simulink model "Extended_Model_1_1"  (R2024a)
settings: Solver=ode15s  StartTime=0.0  StopTime=100  FixedStep=0.0001  MaxStep=0.01  RelTol=1e-3  AbsTol=1e-3  EnableMultiTasking=on
model workspace (MATLAB code in the model file):
  | F_load_x= 2e3; %[N]
  | F_load_y= 1e4; %[N]
  | 
  | d=0.01;   %[m]
  | l=1;      %[m]
  | L=l;      %[m] Node distance
  | H=L*cos(pi/6); %[m] Node distance
  | 
  | Density=7800; %[kg/m^3]
  | E=210;   %[GPa]
  | G=79;    %[GPa]
  | bm=0.01; %[1/s]  Default
  | bk=0.01; %[s] Default
  | 
  | b_rj=1; %[N*m*s/rad] Damp.Coef.Revolut joints
  | 
  | Size_frame=30; %[pixel]
undefined symbols (not defined in the file): F_x, F_y, X, Y, Z
libraries: sm_lib x317, nesl_utility x64, fl_lib x6, simulink x1
(part 1 of 9)
settings Model: NumberOfSteps=100000  Creator=Ing. Štefan Ondočko  LastModifiedBy=Ing. Štefan Ondočko
settings SolverCC: AutoScaleAbsTol=off  MaxZcPerStep=1
settings DataIOCC: LimitDataPoints=on  MaxDataPoints=10000  ReturnWorkspaceOutputs=off
settings OptimizationCC: ReuseModelBlockBuffer=off  LifeSpan=inf
settings DebuggingCC: UnconnectedInputMsg=warning  UnconnectedOutputMsg=warning  UnconnectedLineMsg=warning  AllowSymbolicDim=off  SubsystemReferenceDiagnosticForUnitTest=warning  SFUnexpectedBacktrackingDiag=warning  SFNoUnconditionalDefaultTransitionDiag=warning  SFExecutionAtInitializationDiag=none  ArithmeticOperatorsInVariantConditions=warning
settings ModelReferenceCC: EnableRefExpFcnMdlSchedulingChecks=on
settings SFSimCC: SimUseLocalCustomCode=off  CustomCodeUndefinedFunction=UseInterfaceOnly
settings RTWCC: RTWUseLocalCustomCode=off  GPUComputeCapability=3.5  DLArmComputeVersion=19.05
settings CodeAppCC: StateflowObjectComments=on
settings GRTTargetCC: TargetLangStandard=C89/C90 (ANSI)
settings ConfigComp: CovMetricSettings=dw  CovSaveCumulativeToWorkspaceVar=on  CovSaveSingleToWorkspaceVar=on  CovExternalEMLEnable=off  CovSFcnEnable=off
settings SimscapeCC: SimscapeLogType=all  SimscapeLogSimulationStatistics=on  SimscapeLogDataHistory=10000
settings ExplorerConfigSet: InternalSimMechanicsExplorerSettings="<ExplorerConfiguration><canonicalview>default</canonicalview><AnimationSetting><BasePlaybackSpeed>1.0</BasePlaybackSpeed><PlaybackSpeedFactor>2.0</PlaybackSpeedFactor></AnimationSetting><TilePanel><TileInfo><Tiles Columns=\"1\" Count=\"1\" Rows=\"1\"><Column Weight=\"1\"/><Row Weight=\"1\"/><Tile Height=\"1\" Width=\"1\" X=\"0\" Y=\"0\"/></Tiles></TileInfo><SceneInfo><SceneViewer><BGColor><R>1</R><G>1</G><B>1</B></BGColor><Camera><DoPerspective>off</DoPerspective><Position><X>1.34160017439744395</X><Y>2.43472426416735921</Y><Z>3.19868175252832421</Z></Position><Center><X>1.34160017439744395</X><Y>2.43472426416735921</Y><Z>1.1802899990698279e-08</Z></Center><Up><X>0</X><Y>1</Y><Z>-0</Z></Up><ViewLimDist>1</ViewLimDist><YLim>3.18022072065698147</YLim><XLim>1.97030216076793452</XLim></Camera></SceneViewer></SceneInfo></TilePanel><MechEditorPanel><Cameras/><GfxPanelCameraMap/><VideoCreator><PlaybackSpeedRatio>1.0</PlaybackSpeedRatio><FrameRate>30</FrameRate><VideoFormat>Motion JPEG AVI</VideoFormat><FrameSize>auto</FrameSize></VideoCreator></MechEditorPanel></ExplorerConfiguration>"

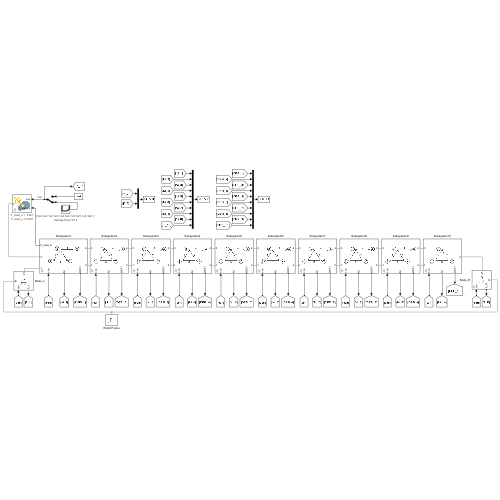
[thumbnail: Simulink's stored preview of the top-level diagram]
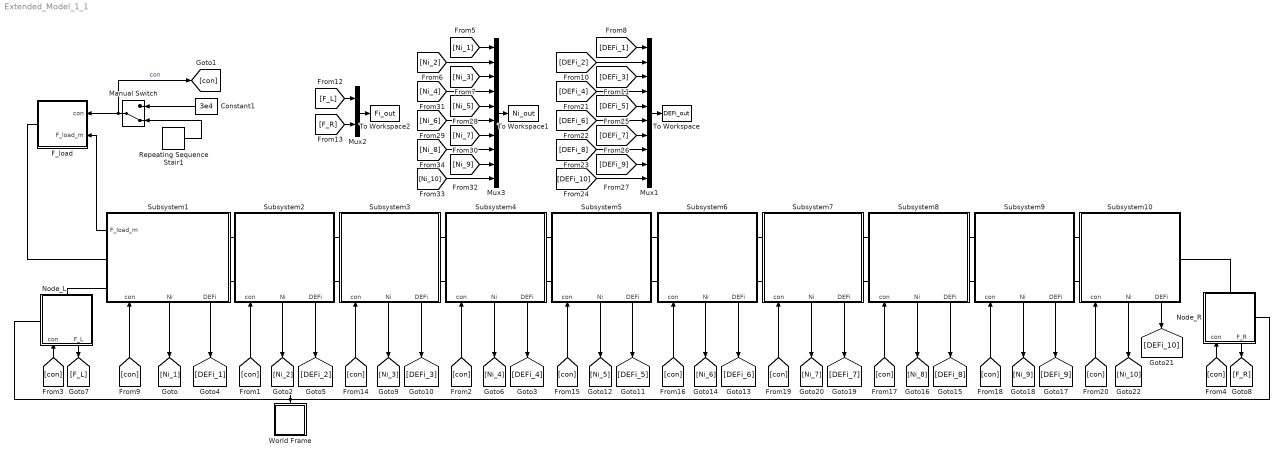
== system Extended_Model_1_1 ==
  Constant1 : Constant  Value=3e4
  F_load : Subsystem  mask{Fx=F_load_x, Fy=F_load_y, F=norm([F_x F_y])}
      mask prompts: Fx "Load Fx (N)"; Fy "Load Fy (N)"; F "Load F (N)"
      settings: AttributesFormatString=|
      | %<Fx> =  2 kN
      | %<Fy> =10 kN
      mask Display: image('D:sila_F.png');
  Manual Switch : ManualSwitch  CurrentSetting=0
  Mux1 : Mux  Inputs=10
  Mux2 : Mux  Inputs=2
  Mux3 : Mux  Inputs=10
  Node_L : Subsystem
      settings: PortSchema="{\"entries\":[{\"content\":{\"sides\":[{\"content\":{\"connectorIds\":[\"LConn1\"]},\"type\":\"ConnectorPlacement.EquallySpacedRectSide\",\"uuid\":\"d437545a-b6cd-405c-92f5-dfd428dd316c\"},{\"content\":{\"side\":\"RIGHT\"},\"type\":\"ConnectorPlacement.EquallySpacedRectSide\",\"uuid\":\"a6c866cb-015a-4ba6-a725-1ad5f0a48a96\"},{\"content\":{\"connectorIds\":[\"In1\",\"Out1\"],\"side\":\"TOP\"},\"type\":\"ConnectorPlacement.EquallySpacedRectSide\",\"uuid\":\"8c34f49c-4b46-4dd5-857b-cc1f00e0721b\"},{\"content\":{\"connectorIds\":[\"RConn1\"],\"side\":\"BOTTOM\"},\"type\":\"ConnectorPlacement.EquallySpacedRectSide\",\"uuid\":\"e1836308-c472-4635-822e-d84e1319bcc1\"}]},\"type\":\"ConnectorPlacement.EquallySpacedConnector\",\"uuid\":\"28d0e514-5749-47ac-8c9d-469c58f8fea4\"}],\"packageUris\":[\"http://schema.mathworks.com/mf0/Connector/R2020b\"],\"version\":\"1.0\"}"
  Node_R : Subsystem  mask{Nod2x=10*L}
      mask prompts: Nod2x "Nod2_offset_x"
      settings: PortSchema="{\"entries\":[{\"content\":{\"sides\":[{\"content\":{},\"type\":\"ConnectorPlacement.EquallySpacedRectSide\",\"uuid\":\"c52cac6f-2005-4bfe-89ae-e2a0406bbacd\"},{\"content\":{\"connectorIds\":[\"RConn1\"],\"side\":\"RIGHT\"},\"type\":\"ConnectorPlacement.EquallySpacedRectSide\",\"uuid\":\"5ceadddb-1bc3-405b-9850-d33e8ff0b50d\"},{\"content\":{\"connectorIds\":[\"In1\",\"Out1\"],\"side\":\"TOP\"},\"type\":\"ConnectorPlacement.EquallySpacedRectSide\",\"uuid\":\"947f3bae-c8fa-4b23-8ea1-709fee7d1677\"},{\"content\":{\"connectorIds\":[\"RConn2\"],\"side\":\"BOTTOM\"},\"type\":\"ConnectorPlacement.EquallySpacedRectSide\",\"uuid\":\"f9cd605e-29e4-49b7-a86d-9958a73b4d00\"}]},\"type\":\"ConnectorPlacement.EquallySpacedConnector\",\"uuid\":\"8856fa92-01df-438d-a79d-88950b3b721b\"}],\"packageUris\":[\"http://schema.mathworks.com/mf0/Connector/R2020b\"],\"version\":\"1.0\"}"
  Repeating Sequence Stair1 : simulink/Sources/Repeating Sequence Stair  OutValues=[1e2 3e2 1e3 3e3 1e4 3e4 1e5 3e5 1e6 3e6 ].'  tsamp=10  OutMin=[]  OutMax=[]  OutDataTypeStr=double  OutputDataTypeScalingMode=double  OutDataType=fixdt(0,8)  ConRadixGroup=Best Precision: Vector-wise  OutScaling=2^-12
      settings: AttributesFormatString=|
      | %<OutValues>
      | SampleTime=%<tsamp> s
  Subsystem1 : Subsystem  mask{Nod2x=-L, Nod3x=-L/2}
      mask prompts: Nod2x "Nod2_offset_x"; Nod3x "Nod3_offset_x"
      settings: PortSchema="{\"entries\":[{\"content\":{\"sides\":[{\"content\":{\"connectorIds\":[\"Out3\",\"LConn1\",\"LConn2\"]},\"type\":\"ConnectorPlacement.EquallySpacedRectSide\",\"uuid\":\"5b691ec6-fd17-4a8f-b07c-565e148aea54\"},{\"content\":{\"connectorIds\":[\"RConn1\",\"RConn2\"],\"side\":\"RIGHT\"},\"type\":\"ConnectorPlacement.EquallySpacedRectSide\",\"uuid\":\"123b4379-6f63-4bac-8b3e-d1a87a3d78c4\"},{\"content\":{\"side\":\"TOP\"},\"type\":\"ConnectorPlacement.EquallySpacedRectSide\",\"uuid\":\"f23bc5ee-4338-4010-a2a0-3e317780f82e\"},{\"content\":{\"connectorIds\":[\"In1\",\"Out1\",\"Out2\"],\"side\":\"BOTTOM\"},\"type\":\"ConnectorPlacement.EquallySpacedRectSide\",\"uuid\":\"f7fe3d2e-1943-42ac-96b9-26c8fbdc1d79\"}]},\"type\":\"ConnectorPlacement.EquallySpacedConnector\",\"uuid\":\"ed714cf3-4128-4128-8bb8-fa1b28911bdc\"}],\"packageUris\":[\"http://schema.mathworks.com/mf0/Connector/R2020b\"],\"version\":\"1.0\"}"
  Subsystem10 : Subsystem  mask{Nod2x=-10*L, Nod3x=-19*L/2}
      mask prompts: Nod2x "Nod2_offset_x"; Nod3x "Nod3_offset_x"
      settings: PortSchema="{\"entries\":[{\"content\":{\"sides\":[{\"content\":{\"connectorIds\":[\"LConn1\",\"LConn2\"]},\"type\":\"ConnectorPlacement.EquallySpacedRectSide\",\"uuid\":\"5b691ec6-fd17-4a8f-b07c-565e148aea54\"},{\"content\":{\"connectorIds\":[\"RConn1\"],\"side\":\"RIGHT\"},\"type\":\"ConnectorPlacement.EquallySpacedRectSide\",\"uuid\":\"123b4379-6f63-4bac-8b3e-d1a87a3d78c4\"},{\"content\":{\"side\":\"TOP\"},\"type\":\"ConnectorPlacement.EquallySpacedRectSide\",\"uuid\":\"f23bc5ee-4338-4010-a2a0-3e317780f82e\"},{\"content\":{\"connectorIds\":[\"In1\",\"Out1\",\"Out2\"],\"side\":\"BOTTOM\"},\"type\":\"ConnectorPlacement.EquallySpacedRectSide\",\"uuid\":\"f7fe3d2e-1943-42ac-96b9-26c8fbdc1d79\"}]},\"type\":\"ConnectorPlacement.EquallySpacedConnector\",\"uuid\":\"ed714cf3-4128-4128-8bb8-fa1b28911bdc\"}],\"packageUris\":[\"http://schema.mathworks.com/mf0/Connector/R2020b\"],\"version\":\"1.0\"}"
  Subsystem2 : Subsystem  mask{Nod2x=-2*L, Nod3x=-3*L/2}
      mask prompts: Nod2x "Nod2_offset_x"; Nod3x "Nod3_offset_x"
      settings: PortSchema="{\"entries\":[{\"content\":{\"sides\":[{\"content\":{\"connectorIds\":[\"LConn1\",\"LConn2\"]},\"type\":\"ConnectorPlacement.EquallySpacedRectSide\",\"uuid\":\"5b691ec6-fd17-4a8f-b07c-565e148aea54\"},{\"content\":{\"connectorIds\":[\"RConn1\",\"RConn2\"],\"side\":\"RIGHT\"},\"type\":\"ConnectorPlacement.EquallySpacedRectSide\",\"uuid\":\"123b4379-6f63-4bac-8b3e-d1a87a3d78c4\"},{\"content\":{\"side\":\"TOP\"},\"type\":\"ConnectorPlacement.EquallySpacedRectSide\",\"uuid\":\"f23bc5ee-4338-4010-a2a0-3e317780f82e\"},{\"content\":{\"connectorIds\":[\"In1\",\"Out1\",\"Out2\"],\"side\":\"BOTTOM\"},\"type\":\"ConnectorPlacement.EquallySpacedRectSide\",\"uuid\":\"f7fe3d2e-1943-42ac-96b9-26c8fbdc1d79\"}]},\"type\":\"ConnectorPlacement.EquallySpacedConnector\",\"uuid\":\"ed714cf3-4128-4128-8bb8-fa1b28911bdc\"}],\"packageUris\":[\"http://schema.mathworks.com/mf0/Connector/R2020b\"],\"version\":\"1.0\"}"
  Subsystem3 : Subsystem  mask{Nod2x=-3*L, Nod3x=-5*L/2}
      mask prompts: Nod2x "Nod2_offset_x"; Nod3x "Nod3_offset_x"
      settings: PortSchema="{\"entries\":[{\"content\":{\"sides\":[{\"content\":{\"connectorIds\":[\"LConn1\",\"LConn2\"]},\"type\":\"ConnectorPlacement.EquallySpacedRectSide\",\"uuid\":\"5b691ec6-fd17-4a8f-b07c-565e148aea54\"},{\"content\":{\"connectorIds\":[\"RConn1\",\"RConn2\"],\"side\":\"RIGHT\"},\"type\":\"ConnectorPlacement.EquallySpacedRectSide\",\"uuid\":\"123b4379-6f63-4bac-8b3e-d1a87a3d78c4\"},{\"content\":{\"side\":\"TOP\"},\"type\":\"ConnectorPlacement.EquallySpacedRectSide\",\"uuid\":\"f23bc5ee-4338-4010-a2a0-3e317780f82e\"},{\"content\":{\"connectorIds\":[\"In1\",\"Out1\",\"Out2\"],\"side\":\"BOTTOM\"},\"type\":\"ConnectorPlacement.EquallySpacedRectSide\",\"uuid\":\"f7fe3d2e-1943-42ac-96b9-26c8fbdc1d79\"}]},\"type\":\"ConnectorPlacement.EquallySpacedConnector\",\"uuid\":\"ed714cf3-4128-4128-8bb8-fa1b28911bdc\"}],\"packageUris\":[\"http://schema.mathworks.com/mf0/Connector/R2020b\"],\"version\":\"1.0\"}"
  Subsystem4 : Subsystem  mask{Nod2x=-4*L, Nod3x=-7*L/2}
      mask prompts: Nod2x "Nod2_offset_x"; Nod3x "Nod3_offset_x"
      settings: PortSchema="{\"entries\":[{\"content\":{\"sides\":[{\"content\":{\"connectorIds\":[\"LConn1\",\"LConn2\"]},\"type\":\"ConnectorPlacement.EquallySpacedRectSide\",\"uuid\":\"5b691ec6-fd17-4a8f-b07c-565e148aea54\"},{\"content\":{\"connectorIds\":[\"RConn1\",\"RConn2\"],\"side\":\"RIGHT\"},\"type\":\"ConnectorPlacement.EquallySpacedRectSide\",\"uuid\":\"123b4379-6f63-4bac-8b3e-d1a87a3d78c4\"},{\"content\":{\"side\":\"TOP\"},\"type\":\"ConnectorPlacement.EquallySpacedRectSide\",\"uuid\":\"f23bc5ee-4338-4010-a2a0-3e317780f82e\"},{\"content\":{\"connectorIds\":[\"In1\",\"Out1\",\"Out2\"],\"side\":\"BOTTOM\"},\"type\":\"ConnectorPlacement.EquallySpacedRectSide\",\"uuid\":\"f7fe3d2e-1943-42ac-96b9-26c8fbdc1d79\"}]},\"type\":\"ConnectorPlacement.EquallySpacedConnector\",\"uuid\":\"ed714cf3-4128-4128-8bb8-fa1b28911bdc\"}],\"packageUris\":[\"http://schema.mathworks.com/mf0/Connector/R2020b\"],\"version\":\"1.0\"}"
  Subsystem5 : Subsystem  mask{Nod2x=-5*L, Nod3x=-9*L/2}
      mask prompts: Nod2x "Nod2_offset_x"; Nod3x "Nod3_offset_x"
      settings: PortSchema="{\"entries\":[{\"content\":{\"sides\":[{\"content\":{\"connectorIds\":[\"LConn1\",\"LConn2\"]},\"type\":\"ConnectorPlacement.EquallySpacedRectSide\",\"uuid\":\"5b691ec6-fd17-4a8f-b07c-565e148aea54\"},{\"content\":{\"connectorIds\":[\"RConn1\",\"RConn2\"],\"side\":\"RIGHT\"},\"type\":\"ConnectorPlacement.EquallySpacedRectSide\",\"uuid\":\"123b4379-6f63-4bac-8b3e-d1a87a3d78c4\"},{\"content\":{\"side\":\"TOP\"},\"type\":\"ConnectorPlacement.EquallySpacedRectSide\",\"uuid\":\"f23bc5ee-4338-4010-a2a0-3e317780f82e\"},{\"content\":{\"connectorIds\":[\"In1\",\"Out1\",\"Out2\"],\"side\":\"BOTTOM\"},\"type\":\"ConnectorPlacement.EquallySpacedRectSide\",\"uuid\":\"f7fe3d2e-1943-42ac-96b9-26c8fbdc1d79\"}]},\"type\":\"ConnectorPlacement.EquallySpacedConnector\",\"uuid\":\"ed714cf3-4128-4128-8bb8-fa1b28911bdc\"}],\"packageUris\":[\"http://schema.mathworks.com/mf0/Connector/R2020b\"],\"version\":\"1.0\"}"
  Subsystem6 : Subsystem  mask{Nod2x=-6*L, Nod3x=-11*L/2}
      mask prompts: Nod2x "Nod2_offset_x"; Nod3x "Nod3_offset_x"
      settings: PortSchema="{\"entries\":[{\"content\":{\"sides\":[{\"content\":{\"connectorIds\":[\"LConn1\",\"LConn2\"]},\"type\":\"ConnectorPlacement.EquallySpacedRectSide\",\"uuid\":\"5b691ec6-fd17-4a8f-b07c-565e148aea54\"},{\"content\":{\"connectorIds\":[\"RConn1\",\"RConn2\"],\"side\":\"RIGHT\"},\"type\":\"ConnectorPlacement.EquallySpacedRectSide\",\"uuid\":\"123b4379-6f63-4bac-8b3e-d1a87a3d78c4\"},{\"content\":{\"side\":\"TOP\"},\"type\":\"ConnectorPlacement.EquallySpacedRectSide\",\"uuid\":\"f23bc5ee-4338-4010-a2a0-3e317780f82e\"},{\"content\":{\"connectorIds\":[\"In1\",\"Out1\",\"Out2\"],\"side\":\"BOTTOM\"},\"type\":\"ConnectorPlacement.EquallySpacedRectSide\",\"uuid\":\"f7fe3d2e-1943-42ac-96b9-26c8fbdc1d79\"}]},\"type\":\"ConnectorPlacement.EquallySpacedConnector\",\"uuid\":\"ed714cf3-4128-4128-8bb8-fa1b28911bdc\"}],\"packageUris\":[\"http://schema.mathworks.com/mf0/Connector/R2020b\"],\"version\":\"1.0\"}"
  Subsystem7 : Subsystem  mask{Nod2x=-7*L, Nod3x=-13*L/2}
      mask prompts: Nod2x "Nod2_offset_x"; Nod3x "Nod3_offset_x"
      settings: PortSchema="{\"entries\":[{\"content\":{\"sides\":[{\"content\":{\"connectorIds\":[\"LConn1\",\"LConn2\"]},\"type\":\"ConnectorPlacement.EquallySpacedRectSide\",\"uuid\":\"5b691ec6-fd17-4a8f-b07c-565e148aea54\"},{\"content\":{\"connectorIds\":[\"RConn1\",\"RConn2\"],\"side\":\"RIGHT\"},\"type\":\"ConnectorPlacement.EquallySpacedRectSide\",\"uuid\":\"123b4379-6f63-4bac-8b3e-d1a87a3d78c4\"},{\"content\":{\"side\":\"TOP\"},\"type\":\"ConnectorPlacement.EquallySpacedRectSide\",\"uuid\":\"f23bc5ee-4338-4010-a2a0-3e317780f82e\"},{\"content\":{\"connectorIds\":[\"In1\",\"Out1\",\"Out2\"],\"side\":\"BOTTOM\"},\"type\":\"ConnectorPlacement.EquallySpacedRectSide\",\"uuid\":\"f7fe3d2e-1943-42ac-96b9-26c8fbdc1d79\"}]},\"type\":\"ConnectorPlacement.EquallySpacedConnector\",\"uuid\":\"ed714cf3-4128-4128-8bb8-fa1b28911bdc\"}],\"packageUris\":[\"http://schema.mathworks.com/mf0/Connector/R2020b\"],\"version\":\"1.0\"}"
  Subsystem8 : Subsystem  mask{Nod2x=-8*L, Nod3x=-15*L/2}
      mask prompts: Nod2x "Nod2_offset_x"; Nod3x "Nod3_offset_x"
      settings: PortSchema="{\"entries\":[{\"content\":{\"sides\":[{\"content\":{\"connectorIds\":[\"LConn1\",\"LConn2\"]},\"type\":\"ConnectorPlacement.EquallySpacedRectSide\",\"uuid\":\"5b691ec6-fd17-4a8f-b07c-565e148aea54\"},{\"content\":{\"connectorIds\":[\"RConn1\",\"RConn2\"],\"side\":\"RIGHT\"},\"type\":\"ConnectorPlacement.EquallySpacedRectSide\",\"uuid\":\"123b4379-6f63-4bac-8b3e-d1a87a3d78c4\"},{\"content\":{\"side\":\"TOP\"},\"type\":\"ConnectorPlacement.EquallySpacedRectSide\",\"uuid\":\"f23bc5ee-4338-4010-a2a0-3e317780f82e\"},{\"content\":{\"connectorIds\":[\"In1\",\"Out1\",\"Out2\"],\"side\":\"BOTTOM\"},\"type\":\"ConnectorPlacement.EquallySpacedRectSide\",\"uuid\":\"f7fe3d2e-1943-42ac-96b9-26c8fbdc1d79\"}]},\"type\":\"ConnectorPlacement.EquallySpacedConnector\",\"uuid\":\"ed714cf3-4128-4128-8bb8-fa1b28911bdc\"}],\"packageUris\":[\"http://schema.mathworks.com/mf0/Connector/R2020b\"],\"version\":\"1.0\"}"
  Subsystem9 : Subsystem  mask{Nod2x=-9*L, Nod3x=-17*L/2}
      mask prompts: Nod2x "Nod2_offset_x"; Nod3x "Nod3_offset_x"
      settings: PortSchema="{\"entries\":[{\"content\":{\"sides\":[{\"content\":{\"connectorIds\":[\"LConn1\",\"LConn2\"]},\"type\":\"ConnectorPlacement.EquallySpacedRectSide\",\"uuid\":\"5b691ec6-fd17-4a8f-b07c-565e148aea54\"},{\"content\":{\"connectorIds\":[\"RConn1\",\"RConn2\"],\"side\":\"RIGHT\"},\"type\":\"ConnectorPlacement.EquallySpacedRectSide\",\"uuid\":\"123b4379-6f63-4bac-8b3e-d1a87a3d78c4\"},{\"content\":{\"side\":\"TOP\"},\"type\":\"ConnectorPlacement.EquallySpacedRectSide\",\"uuid\":\"f23bc5ee-4338-4010-a2a0-3e317780f82e\"},{\"content\":{\"connectorIds\":[\"In1\",\"Out1\",\"Out2\"],\"side\":\"BOTTOM\"},\"type\":\"ConnectorPlacement.EquallySpacedRectSide\",\"uuid\":\"f7fe3d2e-1943-42ac-96b9-26c8fbdc1d79\"}]},\"type\":\"ConnectorPlacement.EquallySpacedConnector\",\"uuid\":\"ed714cf3-4128-4128-8bb8-fa1b28911bdc\"}],\"packageUris\":[\"http://schema.mathworks.com/mf0/Connector/R2020b\"],\"version\":\"1.0\"}"
  To Workspace : ToWorkspace  VariableName=DEFi_out  SampleTime=-1
      settings: Decimation=3
  To Workspace1 : ToWorkspace  VariableName=Ni_out  SampleTime=-1
      settings: Decimation=3
  To Workspace2 : ToWorkspace  VariableName=Fi_out  SampleTime=-1
      settings: Decimation=3
  World Frame : Subsystem
      settings: PortSchema="{\"entries\":[{\"content\":{\"sides\":[{\"content\":{},\"type\":\"ConnectorPlacement.EquallySpacedRectSide\",\"uuid\":\"6a8e21d3-b0b2-4758-a6c8-a7be5ecb73b9\"},{\"content\":{\"side\":\"RIGHT\"},\"type\":\"ConnectorPlacement.EquallySpacedRectSide\",\"uuid\":\"42798d98-bef9-4838-9935-056c1ef1235d\"},{\"content\":{\"connectorIds\":[\"LConn1\"],\"side\":\"TOP\"},\"type\":\"ConnectorPlacement.EquallySpacedRectSide\",\"uuid\":\"7c8f84cf-9fc0-4b00-b00b-766e511bcfac\"}]},\"type\":\"ConnectorPlacement.EquallySpacedConnector\",\"uuid\":\"93a5f294-2ff9-4ffa-a830-6e6e0d522148\"}],\"packageUris\":[\"http://schema.mathworks.com/mf0/Connector/R2020b\"],\"version\":\"1.0\"}"
  wires:
  [con] -> Subsystem1/1(con)
  [con] -> Subsystem2/1(con)
  [con] -> Node_L/1(con)
  [con] -> Node_R/1(con)
  Repeating Sequence Stair1/1 -> Manual Switch/2
  Constant1/1 -> Manual Switch/1
  Manual Switch/1 -> F_load/1(con), [con]  "con"
  Subsystem1/3(F_load_m) -> F_load/2(F_load_m)
  Subsystem1/1(Ni) -> [Ni_1]
  Subsystem2/1(Ni) -> [Ni_2]
  [Ni_1] -> Mux3/1
  [Ni_2] -> Mux3/2
  [Ni_3] -> Mux3/3
  Subsystem1/2(DEFi) -> [DEFi_1]
  Subsystem2/2(DEFi) -> [DEFi_2]
  [DEFi_2] -> Mux1/2
  [DEFi_1] -> Mux1/1
  [DEFi_3] -> Mux1/3
  Node_L/1(F_L) -> [F_L]
  Node_R/1(F_R) -> [F_R]
  [F_R] -> Mux2/2
  [F_L] -> Mux2/1
  Mux2/1 -> To Workspace2/1
  Mux1/1 -> To Workspace/1
  Subsystem3/1(Ni) -> [Ni_3]
  Subsystem3/2(DEFi) -> [DEFi_3]
  [con] -> Subsystem3/1(con)
  Subsystem4/1(Ni) -> [Ni_4]
  [con] -> Subsystem4/1(con)
  Subsystem4/2(DEFi) -> [DEFi_4]
  Subsystem5/1(Ni) -> [Ni_5]
  [con] -> Subsystem5/1(con)
  Subsystem5/2(DEFi) -> [DEFi_5]
  Subsystem6/1(Ni) -> [Ni_6]
  [con] -> Subsystem6/1(con)
  Subsystem6/2(DEFi) -> [DEFi_6]
  [con] -> Subsystem7/1(con)
  Subsystem7/1(Ni) -> [Ni_7]
  Subsystem7/2(DEFi) -> [DEFi_7]
  [con] -> Subsystem8/1(con)
  Subsystem8/2(DEFi) -> [DEFi_8]
  Subsystem8/1(Ni) -> [Ni_8]
  [con] -> Subsystem9/1(con)
  Subsystem9/1(Ni) -> [Ni_9]
  Subsystem9/2(DEFi) -> [DEFi_9]
  [con] -> Subsystem10/1(con)
  Subsystem10/1(Ni) -> [Ni_10]
  Subsystem10/2(DEFi) -> [DEFi_10]
  [DEFi_5] -> Mux1/5
  [DEFi_4] -> Mux1/4
  [DEFi_6] -> Mux1/6
  [DEFi_8] -> Mux1/8
  [DEFi_10] -> Mux1/10
  [DEFi_7] -> Mux1/7
  [DEFi_9] -> Mux1/9
  Mux3/1 -> To Workspace1/1
  [Ni_6] -> Mux3/6
  [Ni_4] -> Mux3/4
  [Ni_5] -> Mux3/5
  [Ni_7] -> Mux3/7
  [Ni_8] -> Mux3/8
  [Ni_10] -> Mux3/10
  [Ni_9] -> Mux3/9
  connections:
  Node_L/LConn1 -- World Frame/LConn1 -- Node_R/RConn1
  Subsystem1/LConn2 -- Node_L/RConn1
  Subsystem1/RConn1 -- Subsystem2/LConn1
  Subsystem1/RConn2 -- Subsystem2/LConn2
  Subsystem10/RConn1 -- Node_R/RConn2
  Subsystem1/LConn1 -- F_load/RConn1
  Subsystem3/LConn2 -- Subsystem2/RConn2
  Subsystem3/LConn1 -- Subsystem2/RConn1
  Subsystem4/LConn1 -- Subsystem3/RConn1
  Subsystem4/LConn2 -- Subsystem3/RConn2
  Subsystem5/LConn1 -- Subsystem4/RConn1
  Subsystem5/LConn2 -- Subsystem4/RConn2
  Subsystem6/LConn1 -- Subsystem5/RConn1
  Subsystem6/LConn2 -- Subsystem5/RConn2
  Subsystem8/LConn1 -- Subsystem7/RConn1
  Subsystem9/LConn1 -- Subsystem8/RConn1
  Subsystem9/LConn2 -- Subsystem8/RConn2
  Subsystem8/LConn2 -- Subsystem7/RConn2
  Subsystem7/LConn1 -- Subsystem6/RConn1
  Subsystem7/LConn2 -- Subsystem6/RConn2
  Subsystem9/RConn1 -- Subsystem10/LConn1
  Subsystem9/RConn2 -- Subsystem10/LConn2

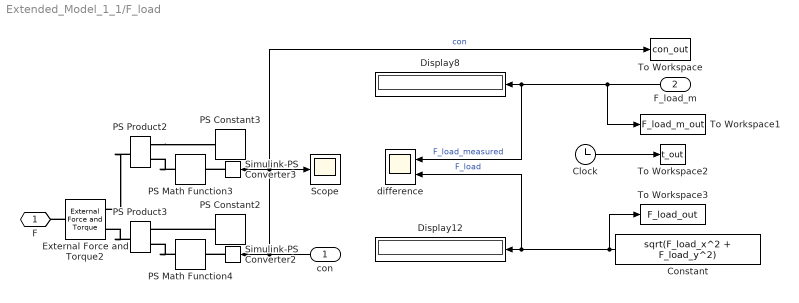
== system Extended_Model_1_1/F_load ==
  con : Inport
  F_load_m : Inport  Port=2
  Clock : Clock
  Constant : Constant  Value=sqrt(F_load_x^2 + F_load_y^2)
  Display12 : Display
      settings: Description=N  AttributesFormatString=%<Description>  Format=long_e
  Display8 : Display
      settings: Description=N  AttributesFormatString=%<Description>  Format=long_e
  External Force and Torque2 : sm_lib/Forces and Torques/External Force and Torque  EnableForceX=on  EnableForceY=on  EnableForceZ=off  EnableForce=off  ForceResolutionFrame=World  EnableTorqueX=off  EnableTorqueY=off  EnableTorqueZ=off  EnableTorque=off  TorqueResolutionFrame=AttachedFrame
  PS Constant2 : fl_lib/Physical Signals/Sources/PS Constant  constant=F_load_y
      settings: AttributesFormatString=%<constant>
  PS Constant3 : fl_lib/Physical Signals/Sources/PS Constant  constant=F_load_x
      settings: AttributesFormatString=%<constant>
  PS Math Function3 : fl_lib/Physical Signals/Functions/PS Math Function  fcn_choice=foundation.enum.math_function.reciprocal  v=1
  PS Math Function4 : fl_lib/Physical Signals/Functions/PS Math Function  fcn_choice=foundation.enum.math_function.reciprocal  v=1
  PS Product2 : fl_lib/Physical Signals/Functions/PS Product
  PS Product3 : fl_lib/Physical Signals/Functions/PS Product
  Scope : Scope
  Simulink-PS Converter2 : nesl_utility/Simulink-PS Converter  PhysicalDomain=network_engine_domain  SubClassName=ps_input  LeftPortType=input  RightPortType=output  PseudoPeriodic=off  Frequencies=[]  NoiseDistribution=none  NoiseParameters=[]  Unit=1  AffineConversion=off  FilteringAndDerivatives=provide  SimscapeFilterOrder=1  InputFilterTimeConstant=0.001  UdotUserProvided=0
  Simulink-PS Converter3 : nesl_utility/Simulink-PS Converter  PhysicalDomain=network_engine_domain  SubClassName=ps_input  LeftPortType=input  RightPortType=output  PseudoPeriodic=off  Frequencies=[]  NoiseDistribution=none  NoiseParameters=[]  Unit=1  AffineConversion=off  FilteringAndDerivatives=provide  SimscapeFilterOrder=1  InputFilterTimeConstant=0.001  UdotUserProvided=0
  To Workspace : ToWorkspace  VariableName=con_out  SampleTime=-1
  To Workspace1 : ToWorkspace  VariableName=F_load_m_out  SampleTime=-1
      settings: Decimation=3
  To Workspace2 : ToWorkspace  VariableName=t_out  SampleTime=-1
      settings: Decimation=3
  To Workspace3 : ToWorkspace  VariableName=F_load_out  SampleTime=-1
      settings: Decimation=3
  difference : Scope  NumInputPorts=2
  F : PMIOPort  Side=Right
  wires:
  F_load_m/1 -> To Workspace1/1, difference/1, Display8/1  "F_load_measured"
  Constant/1 -> To Workspace3/1, Display12/1, difference/2  "F_load"
  Clock/1 -> To Workspace2/1
  con/1 -> To Workspace/1, Scope/1, Simulink-PS Converter3/1, Simulink-PS Converter2/1  "con"
  connections:
  PS Math Function4/RConn1 -- PS Product3/LConn1
  Simulink-PS Converter2/RConn1 -- PS Math Function4/LConn1
  Simulink-PS Converter3/RConn1 -- PS Math Function3/LConn1
  PS Product2/LConn2 -- PS Constant3/RConn1
  PS Math Function3/RConn1 -- PS Product2/LConn1
  PS Constant2/RConn1 -- PS Product3/LConn2
  PS Product2/RConn1 -- External Force and Torque2/LConn1
  PS Product3/RConn1 -- External Force and Torque2/LConn2
  External Force and Torque2/RConn1 -- F/RConn1

== system Extended_Model_1_1/Node_L ==
  note: Node_L
  con : Inport
  Interpreted MATLAB Function : MATLABFcn  Description=u(1:2)  MATLABFcn=u(1:2)
      settings: AttributesFormatString=%<Description>
  PS-Simulink Converter1 : nesl_utility/PS-Simulink Converter  PhysicalDomain=network_engine_domain  SubClassName=ps_output  LeftPortType=input  RightPortType=output  PseudoPeriodic=off  Frequencies=[]  VectorFormat=inherit  Unit=1  AffineConversion=off
  Point : sm_lib/Curves and Surfaces/Point  Description=|  GraphicType=Marker  MarkerShape=Frame  MarkerSize=Size_frame  GraphicVisPropType=SimpleVisualProperties  GraphicDiffuseColor=[1 0 0]  GraphicOpacity=1.0  GraphicSpecularColor=[0.5 0.5 0.5 1.0]  GraphicAmbientColor=[0.15 0.15 0.15 1.0]  GraphicEmissiveColor=[0.0 0.0 0.0 1.0]  GraphicShininess=75
      | Frame
      | visualization
      settings: AttributesFormatString=%<Description>
  Point Cloud : sm_lib/Curves and Surfaces/Point Cloud  Description=|  CoordinatesMatrix=[0 0 0]  CoordinatesMatrixUnits=m  GraphicType=MarkerCloud  GraphicSphereRadius=d/2  GraphicSphereRadiusUnits=m  GraphicVisPropType=SimpleVisualProperties  GraphicDiffuseColor=[0.5 0.5 0.5]  GraphicOpacity=1  GraphicSpecularColor=[0.5 0.5 0.5 1.0]  GraphicAmbientColor=[0.15 0.15 0.15 1.0]  GraphicEmissiveColor=[0.0 0.0 0.0 1.0]  GraphicShininess=75
      | Graphic
      | sphere
      settings: AttributesFormatString=%<Description>
  Product : Product
  Revolute Joint1 : sm_lib/Joints/Revolute Joint  Description=|  JointMode=Normal  CompositeWrenchDir=FollowerOnBase  CompositeWrenchFrame=BaseFrame  SenseConstraintForce=off  SenseConstraintTorque=off  SenseTotalForce=on  SenseTotalTorque=off  PositionTargetSpecify=off  PositionTargetPriority=High  PositionTargetValue=10  PositionTargetValueUnits=deg  VelocityTargetSpecify=off  VelocityTargetPriority=High  VelocityTargetValue=0  VelocityTargetValueUnits=deg/s  EquilibriumPosition=0  EquilibriumPositionUnits=rad  SpringStiffness=0  SpringStiffnessUnits=N*m/rad  DampingCoefficient=b_rj  DampingCoefficientUnits=N*m*s/rad  LowerLimitSpecify=off  LowerLimitBound=-90  LowerLimitBoundUnits=deg  LowerLimitStiffness=1e4  LowerLimitStiffnessUnits=N*m/deg  LowerLimitDamping=10  LowerLimitDampingUnits=N*m/(deg/s)  LowerLimitTransitionRegionWidth=0.1  LowerLimitTransitionRegionWidthUnits=deg  UpperLimitSpecify=off  UpperLimitBound=90  UpperLimitBoundUnits=deg  UpperLimitStiffness=1e4  UpperLimitStiffnessUnits=N*m/deg  UpperLimitDamping=10  UpperLimitDampingUnits=N*m/(deg/s)  UpperLimitTransitionRegionWidth=0.1  UpperLimitTransitionRegionWidthUnits=deg  TorqueActuationMode=NoTorque  MotionActuationMode=ComputedMotion  SensePosition=off  SenseVelocity=off  SenseAcceleration=off  SenseTorqueForce=off  SenseLowerLimitTorqueForce=off  SenseUpperLimitTorqueForce=off
      | Total force
      | sensing
  B : PMIOPort  Side=Left
  F1 : PMIOPort  Port=2  Side=Right
  F_L : Outport
  wires:
  PS-Simulink Converter1/1 -> Interpreted MATLAB Function/1
  Interpreted MATLAB Function/1 -> Product/1
  Product/1 -> F_L/1
  con/1 -> Product/2
  connections:
  Point Cloud/LConn1 -- Revolute Joint1/RConn1 -- F1/RConn1
  PS-Simulink Converter1/LConn1 -- Revolute Joint1/RConn2
  Revolute Joint1/LConn1 -- Point/LConn1 -- B/RConn1

== system Extended_Model_1_1/Node_R ==
  note: Node_R
  con : Inport
  Interpreted MATLAB Function : MATLABFcn  Description=u(1:2)  MATLABFcn=u(1:2)
      settings: AttributesFormatString=%<Description>
  PS-Simulink Converter1 : nesl_utility/PS-Simulink Converter  PhysicalDomain=network_engine_domain  SubClassName=ps_output  LeftPortType=input  RightPortType=output  PseudoPeriodic=off  Frequencies=[]  VectorFormat=inherit  Unit=1  AffineConversion=off
  Point Cloud2 : sm_lib/Curves and Surfaces/Point Cloud  Description=|  CoordinatesMatrix=[0 0 0]  CoordinatesMatrixUnits=m  GraphicType=MarkerCloud  GraphicSphereRadius=d/2  GraphicSphereRadiusUnits=m  GraphicVisPropType=SimpleVisualProperties  GraphicDiffuseColor=[0.5 0.5 0.5]  GraphicOpacity=1  GraphicSpecularColor=[0.5 0.5 0.5 1.0]  GraphicAmbientColor=[0.15 0.15 0.15 1.0]  GraphicEmissiveColor=[0.0 0.0 0.0 1.0]  GraphicShininess=75
      | Graphic
      | sphere
      settings: AttributesFormatString=%<Description>
  Point1 : sm_lib/Curves and Surfaces/Point  Description=|  GraphicType=Marker  MarkerShape=Frame  MarkerSize=Size_frame  GraphicVisPropType=SimpleVisualProperties  GraphicDiffuseColor=[1 0 0]  GraphicOpacity=1.0  GraphicSpecularColor=[0.5 0.5 0.5 1.0]  GraphicAmbientColor=[0.15 0.15 0.15 1.0]  GraphicEmissiveColor=[0.0 0.0 0.0 1.0]  GraphicShininess=75
      | Frame
      | visualization
      settings: AttributesFormatString=%<Description>
  Product : Product
  Revolute Joint : sm_lib/Joints/Revolute Joint  JointMode=Normal  CompositeWrenchDir=FollowerOnBase  CompositeWrenchFrame=BaseFrame  SenseConstraintForce=off  SenseConstraintTorque=off  SenseTotalForce=on  SenseTotalTorque=off  PositionTargetSpecify=off  PositionTargetPriority=High  PositionTargetValue=0  PositionTargetValueUnits=deg  VelocityTargetSpecify=off  VelocityTargetPriority=High  VelocityTargetValue=0  VelocityTargetValueUnits=deg/s  EquilibriumPosition=0  EquilibriumPositionUnits=rad  SpringStiffness=0  SpringStiffnessUnits=N*m/rad  DampingCoefficient=b_rj  DampingCoefficientUnits=N*m*s/rad  LowerLimitSpecify=off  LowerLimitBound=-90  LowerLimitBoundUnits=deg  LowerLimitStiffness=1e4  LowerLimitStiffnessUnits=N*m/deg  LowerLimitDamping=10  LowerLimitDampingUnits=N*m/(deg/s)  LowerLimitTransitionRegionWidth=0.1  LowerLimitTransitionRegionWidthUnits=deg  UpperLimitSpecify=off  UpperLimitBound=90  UpperLimitBoundUnits=deg  UpperLimitStiffness=1e4  UpperLimitStiffnessUnits=N*m/deg  UpperLimitDamping=10  UpperLimitDampingUnits=N*m/(deg/s)  UpperLimitTransitionRegionWidth=0.1  UpperLimitTransitionRegionWidthUnits=deg  TorqueActuationMode=NoTorque  MotionActuationMode=ComputedMotion  SensePosition=off  SenseVelocity=off  SenseAcceleration=off  SenseTorqueForce=off  SenseLowerLimitTorqueForce=off  SenseUpperLimitTorqueForce=off
  Rigid Transform1 : sm_lib/Frames and Transforms/Rigid Transform  Description=Offset  RotationMethod=None  FollAlignAxisA=+X  BaseAlignAxisA=+Y  FollAlignAxisB=+Y  BaseAlignAxisB=+Z  RotationStandardAxis=+Z  RotationAngle=0.0  RotationAngleUnits=deg  RotationArbitraryAxis=[0 0 1]  RotationSequenceAxes=FollowerAxes  RotationSequence=XYX  RotationSequenceAngles=[0 0 0]  RotationSequenceAnglesUnits=deg  RotationMatrix=[1 0 0; 0 1 0; 0 0 1]  Quaternion=[1 0 0 0]  TranslationMethod=Cartesian  TranslationCartesianOffset=[Nod2x 0 0]  TranslationCartesianOffsetUnits=m  TranslationStandardAxis=+Z  TranslationStandardOffset=0  TranslationStandardOffsetUnits=m  TranslationROffset=0  TranslationROffsetUnits=m  TranslationThetaOffset=0  TranslationThetaOffsetUnits=deg  TranslationZOffset=0  TranslationZOffsetUnits=m
      settings: AttributesFormatString=|
      | %<Description>
      | %<TranslationCartesianOffset> %<TranslationCartesianOffsetUnits>
  B : PMIOPort  Side=Right
  F1 : PMIOPort  Port=2  Side=Right
  F_R : Outport
  wires:
  PS-Simulink Converter1/1 -> Interpreted MATLAB Function/1
  con/1 -> Product/2
  Product/1 -> F_R/1
  Interpreted MATLAB Function/1 -> Product/1
  connections:
  F1/RConn1 -- Point Cloud2/LConn1 -- Revolute Joint/RConn1
  Rigid Transform1/RConn1 -- Revolute Joint/LConn1 -- Point1/LConn1
  Revolute Joint/RConn2 -- PS-Simulink Converter1/LConn1
  Rigid Transform1/LConn1 -- B/RConn1

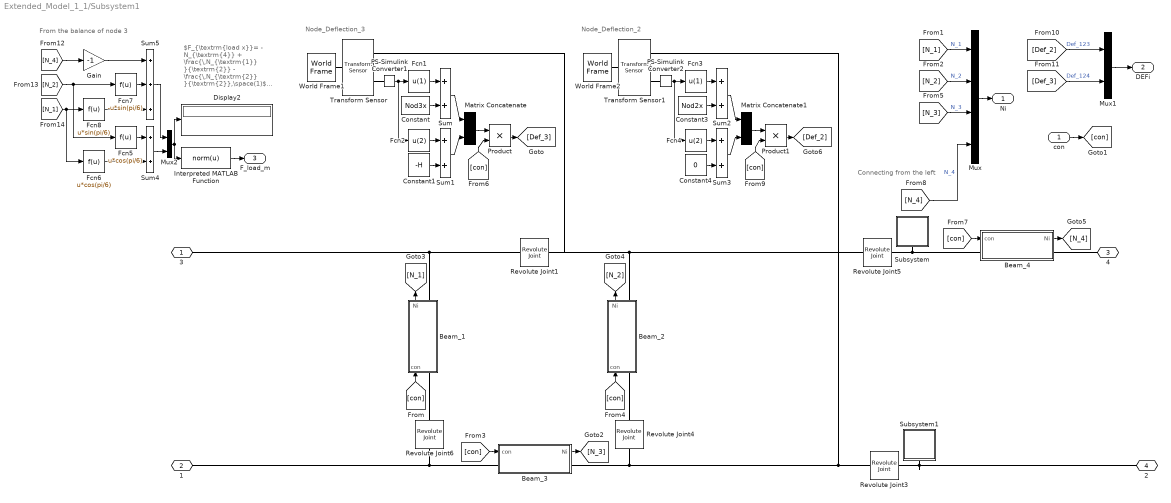
== system Extended_Model_1_1/Subsystem1 ==
  note: Connecting from the left
  note: Node_Deflection_3
  note: Node_Deflection_2
  note: $F_{\textrm{load x}}= - N_{\textrm{4}} + \frac{\,N_{\textrm{1}} }{\textrm{2}} - \frac{\,N_{\textrm{2}} }{\textrm{2}},\space(1)$
      | $F_{\textrm{load y}}=\frac{\sqrt{3}\,N_1 }{2} + \frac{\sqrt{3}\,N_2 }{2},\space(2)$
  note: From the balance of node 3
  con : Inport
  Beam_1 : Subsystem
  Beam_2 : Subsystem
  Beam_3 : Subsystem
  Beam_4 : Subsystem
  Constant : Constant  Value=Nod3x
  Constant1 : Constant  Value=-H
  Constant3 : Constant  Value=Nod2x
  Constant4 : Constant  Value=0
  Display2 : Display
      settings: Description=N  AttributesFormatString=%<Description>  Format=long_e
  Fcn1 : Fcn  Expr=u(1)
  Fcn2 : Fcn  Expr=u(2)
  Fcn3 : Fcn  Expr=u(1)
  Fcn4 : Fcn  Expr=u(2)
  Fcn5 : Fcn  Description=-u/sqrt(2)  Expr=u*cos(pi/6)
      settings: AttributesFormatString=%<Expr>
  Fcn6 : Fcn  Description=-u/sqrt(2)  Expr=u*cos(pi/6)
      settings: AttributesFormatString=%<Expr>
  Fcn7 : Fcn  Description=-u/sqrt(2)  Expr=-u*sin(pi/6)
      settings: AttributesFormatString=%<Expr>
  Fcn8 : Fcn  Description=-u/sqrt(2)  Expr=u*sin(pi/6)
      settings: AttributesFormatString=%<Expr>
  Gain : Gain  Gain=-1
  Interpreted MATLAB Function : MATLABFcn  Description=Norm  MATLABFcn=norm(u)
      settings: AttributesFormatString=%<Description>
  Matrix Concatenate : Concatenate  ConcatenateDimension=2
      settings: AttributesFormatString=%<Description>
  Matrix Concatenate1 : Concatenate  ConcatenateDimension=2
      settings: AttributesFormatString=%<Description>
  Mux : Mux
  Mux1 : Mux  Inputs=2
  Mux2 : Mux  Inputs=2
  PS-Simulink Converter1 : nesl_utility/PS-Simulink Converter  PhysicalDomain=network_engine_domain  SubClassName=ps_output  LeftPortType=input  RightPortType=output  PseudoPeriodic=off  Frequencies=[]  VectorFormat=inherit  Unit=1  AffineConversion=off
  PS-Simulink Converter2 : nesl_utility/PS-Simulink Converter  PhysicalDomain=network_engine_domain  SubClassName=ps_output  LeftPortType=input  RightPortType=output  PseudoPeriodic=off  Frequencies=[]  VectorFormat=inherit  Unit=1  AffineConversion=off
  Product : Product
  Product1 : Product
  Revolute Joint1 : sm_lib/Joints/Revolute Joint  JointMode=Normal  CompositeWrenchDir=FollowerOnBase  CompositeWrenchFrame=BaseFrame  SenseConstraintForce=off  SenseConstraintTorque=off  SenseTotalForce=off  SenseTotalTorque=off  PositionTargetSpecify=on  PositionTargetPriority=Low  PositionTargetValue=pi/3  PositionTargetValueUnits=rad  VelocityTargetSpecify=off  VelocityTargetPriority=High  VelocityTargetValue=0  VelocityTargetValueUnits=deg/s  EquilibriumPosition=0  EquilibriumPositionUnits=rad  SpringStiffness=0  SpringStiffnessUnits=N*m/rad  DampingCoefficient=b_rj  DampingCoefficientUnits=N*m*s/rad  LowerLimitSpecify=off  LowerLimitBound=-90  LowerLimitBoundUnits=deg  LowerLimitStiffness=1e4  LowerLimitStiffnessUnits=N*m/deg  LowerLimitDamping=10  LowerLimitDampingUnits=N*m/(deg/s)  LowerLimitTransitionRegionWidth=0.1  LowerLimitTransitionRegionWidthUnits=deg  UpperLimitSpecify=off  UpperLimitBound=90  UpperLimitBoundUnits=deg  UpperLimitStiffness=1e4  UpperLimitStiffnessUnits=N*m/deg  UpperLimitDamping=10  UpperLimitDampingUnits=N*m/(deg/s)  UpperLimitTransitionRegionWidth=0.1  UpperLimitTransitionRegionWidthUnits=deg  TorqueActuationMode=NoTorque  MotionActuationMode=ComputedMotion  SensePosition=off  SenseVelocity=off  SenseAcceleration=off  SenseTorqueForce=off  SenseLowerLimitTorqueForce=off  SenseUpperLimitTorqueForce=off
      settings: AttributesFormatString=%<PositionTargetValue>
  Revolute Joint3 : sm_lib/Joints/Revolute Joint  JointMode=Normal  CompositeWrenchDir=FollowerOnBase  CompositeWrenchFrame=BaseFrame  SenseConstraintForce=off  SenseConstraintTorque=off  SenseTotalForce=off  SenseTotalTorque=off  PositionTargetSpecify=on  PositionTargetPriority=Low  PositionTargetValue=0  PositionTargetValueUnits=rad  VelocityTargetSpecify=off  VelocityTargetPriority=High  VelocityTargetValue=0  VelocityTargetValueUnits=deg/s  EquilibriumPosition=0  EquilibriumPositionUnits=rad  SpringStiffness=0  SpringStiffnessUnits=N*m/rad  DampingCoefficient=b_rj  DampingCoefficientUnits=N*m*s/rad  LowerLimitSpecify=off  LowerLimitBound=-90  LowerLimitBoundUnits=deg  LowerLimitStiffness=1e4  LowerLimitStiffnessUnits=N*m/deg  LowerLimitDamping=10  LowerLimitDampingUnits=N*m/(deg/s)  LowerLimitTransitionRegionWidth=0.1  LowerLimitTransitionRegionWidthUnits=deg  UpperLimitSpecify=off  UpperLimitBound=90  UpperLimitBoundUnits=deg  UpperLimitStiffness=1e4  UpperLimitStiffnessUnits=N*m/deg  UpperLimitDamping=10  UpperLimitDampingUnits=N*m/(deg/s)  UpperLimitTransitionRegionWidth=0.1  UpperLimitTransitionRegionWidthUnits=deg  TorqueActuationMode=NoTorque  MotionActuationMode=ComputedMotion  SensePosition=off  SenseVelocity=off  SenseAcceleration=off  SenseTorqueForce=off  SenseLowerLimitTorqueForce=off  SenseUpperLimitTorqueForce=off
      settings: AttributesFormatString=%<PositionTargetValue>
  Revolute Joint4 : sm_lib/Joints/Revolute Joint  JointMode=Normal  CompositeWrenchDir=FollowerOnBase  CompositeWrenchFrame=BaseFrame  SenseConstraintForce=off  SenseConstraintTorque=off  SenseTotalForce=off  SenseTotalTorque=off  PositionTargetSpecify=off  PositionTargetPriority=High  PositionTargetValue=0  PositionTargetValueUnits=deg  VelocityTargetSpecify=off  VelocityTargetPriority=High  VelocityTargetValue=0  VelocityTargetValueUnits=deg/s  EquilibriumPosition=0  EquilibriumPositionUnits=rad  SpringStiffness=0  SpringStiffnessUnits=N*m/rad  DampingCoefficient=b_rj  DampingCoefficientUnits=N*m*s/rad  LowerLimitSpecify=off  LowerLimitBound=-90  LowerLimitBoundUnits=deg  LowerLimitStiffness=1e4  LowerLimitStiffnessUnits=N*m/deg  LowerLimitDamping=10  LowerLimitDampingUnits=N*m/(deg/s)  LowerLimitTransitionRegionWidth=0.1  LowerLimitTransitionRegionWidthUnits=deg  UpperLimitSpecify=off  UpperLimitBound=90  UpperLimitBoundUnits=deg  UpperLimitStiffness=1e4  UpperLimitStiffnessUnits=N*m/deg  UpperLimitDamping=10  UpperLimitDampingUnits=N*m/(deg/s)  UpperLimitTransitionRegionWidth=0.1  UpperLimitTransitionRegionWidthUnits=deg  TorqueActuationMode=NoTorque  MotionActuationMode=ComputedMotion  SensePosition=off  SenseVelocity=off  SenseAcceleration=off  SenseTorqueForce=off  SenseLowerLimitTorqueForce=off  SenseUpperLimitTorqueForce=off
  Revolute Joint5 : sm_lib/Joints/Revolute Joint  JointMode=Normal  CompositeWrenchDir=FollowerOnBase  CompositeWrenchFrame=BaseFrame  SenseConstraintForce=off  SenseConstraintTorque=off  SenseTotalForce=off  SenseTotalTorque=off  PositionTargetSpecify=on  PositionTargetPriority=Low  PositionTargetValue=-4*pi/6  PositionTargetValueUnits=rad  VelocityTargetSpecify=off  VelocityTargetPriority=High  VelocityTargetValue=0  VelocityTargetValueUnits=deg/s  EquilibriumPosition=0  EquilibriumPositionUnits=rad  SpringStiffness=0  SpringStiffnessUnits=N*m/rad  DampingCoefficient=b_rj  DampingCoefficientUnits=N*m*s/rad  LowerLimitSpecify=off  LowerLimitBound=-90  LowerLimitBoundUnits=deg  LowerLimitStiffness=1e4  LowerLimitStiffnessUnits=N*m/deg  LowerLimitDamping=10  LowerLimitDampingUnits=N*m/(deg/s)  LowerLimitTransitionRegionWidth=0.1  LowerLimitTransitionRegionWidthUnits=deg  UpperLimitSpecify=off  UpperLimitBound=90  UpperLimitBoundUnits=deg  UpperLimitStiffness=1e4  UpperLimitStiffnessUnits=N*m/deg  UpperLimitDamping=10  UpperLimitDampingUnits=N*m/(deg/s)  UpperLimitTransitionRegionWidth=0.1  UpperLimitTransitionRegionWidthUnits=deg  TorqueActuationMode=NoTorque  MotionActuationMode=ComputedMotion  SensePosition=off  SenseVelocity=off  SenseAcceleration=off  SenseTorqueForce=off  SenseLowerLimitTorqueForce=off  SenseUpperLimitTorqueForce=off
      settings: AttributesFormatString=%<PositionTargetValue>
  Revolute Joint6 : sm_lib/Joints/Revolute Joint  JointMode=Normal  CompositeWrenchDir=FollowerOnBase  CompositeWrenchFrame=BaseFrame  SenseConstraintForce=off  SenseConstraintTorque=off  SenseTotalForce=off  SenseTotalTorque=off  PositionTargetSpecify=on  PositionTargetPriority=Low  PositionTargetValue=pi/3  PositionTargetValueUnits=rad  VelocityTargetSpecify=off  VelocityTargetPriority=High  VelocityTargetValue=0  VelocityTargetValueUnits=deg/s  EquilibriumPosition=0  EquilibriumPositionUnits=rad  SpringStiffness=0  SpringStiffnessUnits=N*m/rad  DampingCoefficient=b_rj  DampingCoefficientUnits=N*m*s/rad  LowerLimitSpecify=off  LowerLimitBound=-90  LowerLimitBoundUnits=deg  LowerLimitStiffness=1e4  LowerLimitStiffnessUnits=N*m/deg  LowerLimitDamping=10  LowerLimitDampingUnits=N*m/(deg/s)  LowerLimitTransitionRegionWidth=0.1  LowerLimitTransitionRegionWidthUnits=deg  UpperLimitSpecify=off  UpperLimitBound=90  UpperLimitBoundUnits=deg  UpperLimitStiffness=1e4  UpperLimitStiffnessUnits=N*m/deg  UpperLimitDamping=10  UpperLimitDampingUnits=N*m/(deg/s)  UpperLimitTransitionRegionWidth=0.1  UpperLimitTransitionRegionWidthUnits=deg  TorqueActuationMode=NoTorque  MotionActuationMode=ComputedMotion  SensePosition=off  SenseVelocity=off  SenseAcceleration=off  SenseTorqueForce=off  SenseLowerLimitTorqueForce=off  SenseUpperLimitTorqueForce=off
      settings: AttributesFormatString=%<PositionTargetValue>
  Subsystem : Subsystem
  Subsystem1 : Subsystem
  Sum{,1..3} (4 alike) : Sum  Inputs=2
  Sum4 : Sum
  Sum5 : Sum  Inputs=3
  Transform Sensor : sm_lib/Frames and Transforms/Transform Sensor  Description=|  MeasurementFrame=World  RotationSequence=XYX  SenseAngle=off  SenseAxis=off  SenseQ=off  SenseR=off  SenseRotationSequence=off  SenseOmegaX=off  SenseOmegaY=off  SenseOmegaZ=off  SenseOmega=off  SenseQDot=off  SenseRDot=off  SenseRotationSequenceDot=off  SenseAlphaX=off  SenseAlphaY=off  SenseAlphaZ=off  SenseAlpha=off  SenseQDDot=off  SenseRDDot=off  SenseX=off  SenseY=off  SenseZ=off  SenseXYZ=on  SenseRad=off  SenseAzim=off  SenseDist=off  SenseInc=off  SenseXDot=off  SenseYDot=off  SenseZDot=off  SenseXYZDot=off  SenseRadDot=off  SenseAzimDot=off  SenseDistDot=off  SenseIncDot=off  SenseXDDot=off  SenseYDDot=off  SenseZDDot=off  SenseXYZDDot=off  SenseRadDDot=off  SenseAzimDDot=off  SenseDistDDot=off  SenseIncDDot=off
      | Translation
      | [x, y, z]
      settings: AttributesFormatString=%<Description>
  Transform Sensor1 : sm_lib/Frames and Transforms/Transform Sensor  Description=|  MeasurementFrame=World  RotationSequence=XYX  SenseAngle=off  SenseAxis=off  SenseQ=off  SenseR=off  SenseRotationSequence=off  SenseOmegaX=off  SenseOmegaY=off  SenseOmegaZ=off  SenseOmega=off  SenseQDot=off  SenseRDot=off  SenseRotationSequenceDot=off  SenseAlphaX=off  SenseAlphaY=off  SenseAlphaZ=off  SenseAlpha=off  SenseQDDot=off  SenseRDDot=off  SenseX=off  SenseY=off  SenseZ=off  SenseXYZ=on  SenseRad=off  SenseAzim=off  SenseDist=off  SenseInc=off  SenseXDot=off  SenseYDot=off  SenseZDot=off  SenseXYZDot=off  SenseRadDot=off  SenseAzimDot=off  SenseDistDot=off  SenseIncDot=off  SenseXDDot=off  SenseYDDot=off  SenseZDDot=off  SenseXYZDDot=off  SenseRadDDot=off  SenseAzimDDot=off  SenseDistDDot=off  SenseIncDDot=off
      | Translation
      | [x, y, z]
      settings: AttributesFormatString=%<Description>
  World Frame1 : sm_lib/Frames and Transforms/World Frame
  World Frame2 : sm_lib/Frames and Transforms/World Frame
  3 : PMIOPort  Side=Left
  1 : PMIOPort  Port=2  Side=Left
  4 : PMIOPort  Port=3  Side=Right
  2 : PMIOPort  Port=4  Side=Right
  Ni : Outport
  DEFi : Outport  Port=2
  F_load_m : Outport  Port=3
  wires:
  Sum2/1 -> Matrix Concatenate1/1
  Constant1/1 -> Sum1/2
  PS-Simulink Converter2/1 -> Fcn4/1, Fcn3/1
  Matrix Concatenate1/1 -> Product1/1
  [N_2] -> Mux/2  "N_2"
  Fcn1/1 -> Sum/1
  PS-Simulink Converter1/1 -> Fcn2/1, Fcn1/1
  [N_4] -> Mux/4  "N_4"
  Mux1/1 -> DEFi/1
  Beam_1/1(Ni) -> [N_1]
  [con] -> Beam_1/1(con)
  Beam_3/1(Ni) -> [N_3]
  [Def_2] -> Mux1/1  "Def_123"
  Constant/1 -> Sum/2
  [con] -> Product1/2
  [con] -> Beam_2/1(con)
  Fcn4/1 -> Sum3/1
  Beam_4/1(Ni) -> [N_4]
  Sum/1 -> Matrix Concatenate/1
  [con] -> Product/2
  Sum1/1 -> Matrix Concatenate/2
  Matrix Concatenate/1 -> Product/1
  Mux/1 -> Ni/1
  [Def_3] -> Mux1/2  "Def_124"
  Sum3/1 -> Matrix Concatenate1/2
  Product/1 -> [Def_3]
  Fcn2/1 -> Sum1/1
  Constant3/1 -> Sum2/2
  Beam_2/1(Ni) -> [N_2]
  Constant4/1 -> Sum3/2
  Product1/1 -> [Def_2]
  Fcn3/1 -> Sum2/1
  [con] -> Beam_4/1(con)
  con/1 -> [con]
  [con] -> Beam_3/1(con)
  [N_1] -> Mux/1  "N_1"
  [N_3] -> Mux/3  "N_3"
  [N_4] -> Gain/1
  Gain/1 -> Sum5/1
  Interpreted MATLAB Function/1 -> F_load_m/1
  Fcn6/1 -> Sum4/2
  Fcn5/1 -> Sum4/1
  Mux2/1 -> Display2/1, Interpreted MATLAB Function/1
  [N_2] -> Fcn7/1, Fcn5/1
  Fcn7/1 -> Sum5/2
  Sum5/1 -> Mux2/1
  Sum4/1 -> Mux2/2
  Fcn8/1 -> Sum5/3
  [N_1] -> Fcn8/1, Fcn6/1
  connections:
  Subsystem1/LConn1 -- Revolute Joint3/RConn1 -- 2/RConn1
  Revolute Joint6/RConn1 -- Beam_1/LConn1
  World Frame2/RConn1 -- Transform Sensor1/LConn1
  Revolute Joint3/LConn1 -- Beam_3/RConn1 -- Revolute Joint4/LConn1 -- Transform Sensor1/RConn1
  Revolute Joint1/LConn1 -- 3/RConn1 -- Beam_1/RConn1
  Revolute Joint5/RConn1 -- Beam_4/LConn1 -- Subsystem/LConn1
  PS-Simulink Converter2/LConn1 -- Transform Sensor1/RConn2
  Revolute Joint4/RConn1 -- Beam_2/LConn1
  Revolute Joint5/LConn1 -- Beam_2/RConn1 -- Revolute Joint1/RConn1 -- Transform Sensor/RConn1
  World Frame1/RConn1 -- Transform Sensor/LConn1
  Beam_4/RConn1 -- 4/RConn1
  Revolute Joint6/LConn1 -- Beam_3/LConn1 -- 1/RConn1
  PS-Simulink Converter1/LConn1 -- Transform Sensor/RConn2
